simulink model "wzorzec_nasze"  (R2021b)
settings: Solver=ode5  StartTime=0.0  StopTime=20  FixedStep=0.01  RelTol=1e-3
settings Model: SimulationMode=external  ExtModeTrigDuration=100000  Creator=STUDENT  LastModifiedBy=STUDENT
settings SolverCC: AlgebraicLoopSolver=TrustRegion  DecoupledContinuousIntegration=on  MinimalZcImpactIntegration=on
settings DataIOCC: ReturnWorkspaceOutputs=off
settings DebuggingCC: PregeneratedLibrarySubsystemCodeDiagnostic=none  SFMachineParentedDataDiag=warning  ArithmeticOperatorsInVariantConditions=warning
settings SFSimCC: SimUseLocalCustomCode=off  CustomCodeUndefinedFunction=UseInterfaceOnly
settings RTWCC: Description=Simulink Desktop Real-Time  SystemTargetFile=sldrt.tlc  TemplateMakefile=sldrt.tmf  RTWUseLocalCustomCode=off  RTWCompilerOptimization=on
settings CodeAppCC: MaxIdLength=95
settings SimulinkDesktopRealTimeCC: TargetPreCompLibLocation=C:\apps\MATLAB\R2021b\toolbox\sldrt\lib\win64

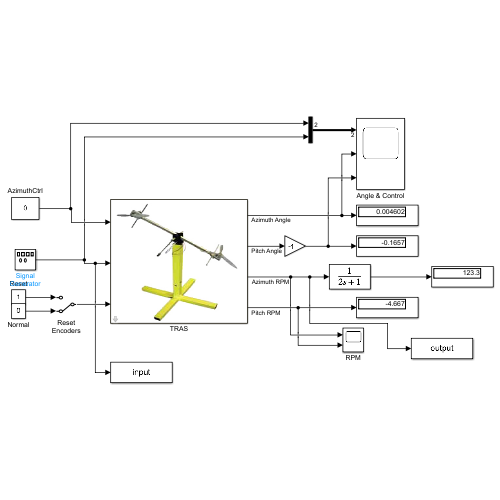
[thumbnail: Simulink's stored preview of the top-level diagram]
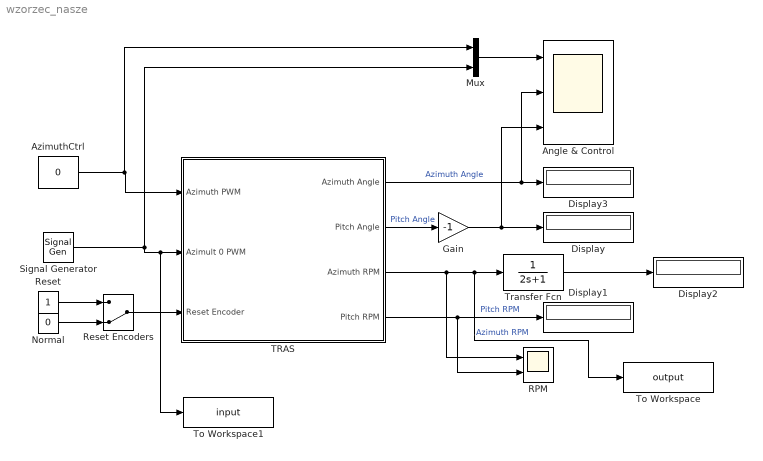
== system wzorzec_nasze ==
  Angle & Control : Scope  NumInputPorts=3
  AzimuthCtrl : Constant  Value=0
  Display{,1..3} (4 alike) : Display
  Gain : Gain  Gain=-1
  Mux : Mux  Inputs=2
  Normal : Constant  Value=0
  RPM : Scope  NumInputPorts=2
  Reset : Constant
  Reset Encoders : ManualSwitch  CurrentSetting=0
  Signal Generator : SignalGenerator  WaveForm=square  Amplitude=0.6  Frequency=0.5
  TRAS : Subsystem  mask{BaseAddress=57088, T0=0.01}
      mask prompts: BaseAddress "Base Address:"; T0 "Sampling Period:"
      mask Display: image('TRAS.JPG')
  To Workspace : ToWorkspace  VariableName=output  SaveFormat=Structure With Time  SampleTime=0.01
  To Workspace1 : ToWorkspace  VariableName=input  SaveFormat=Structure With Time  SampleTime=0.01
  Transfer Fcn : TransferFcn  Denominator=[2 1]
  wires:
  Reset/1 -> Reset Encoders/1
  TRAS/3(Azimuth RPM) -> To Workspace/1, Transfer Fcn/1, RPM/1  "Azimuth RPM"
  TRAS/1(Azimuth Angle) -> Angle & Control/2, Display3/1  "Azimuth Angle"
  TRAS/4(Pitch RPM) -> RPM/2, Display1/1  "Pitch RPM"
  Normal/1 -> Reset Encoders/2
  Reset Encoders/1 -> TRAS/3(Reset Encoder)
  TRAS/2(Pitch Angle) -> Gain/1  "Pitch Angle"
  Gain/1 -> Angle & Control/3, Display/1
  Mux/1 -> Angle & Control/1
  AzimuthCtrl/1 -> Mux/1, TRAS/1(Azimuth PWM)
  Transfer Fcn/1 -> Display2/1
  Signal Generator/1 -> To Workspace1/1, TRAS/2(Azimult 0 PWM), Mux/2

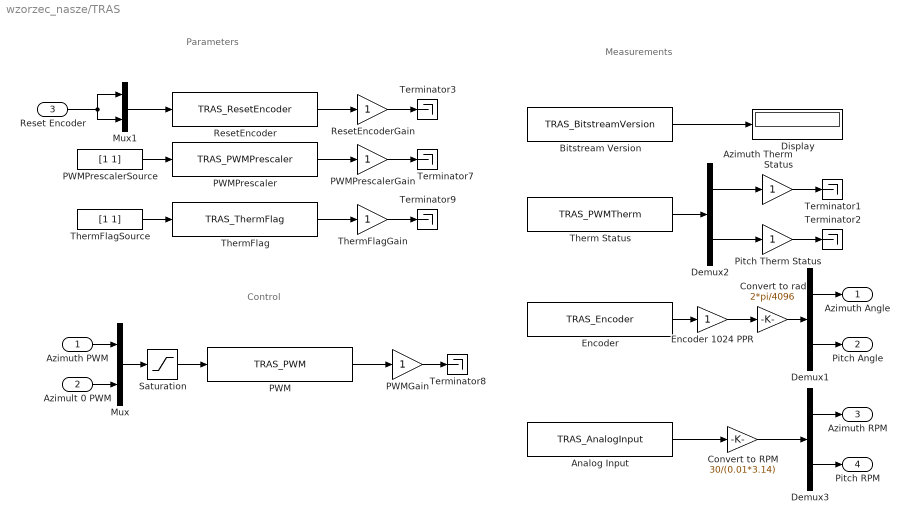
== system wzorzec_nasze/TRAS ==
  note: Parameters
  note: Control
  note: Measurements
  Azimuth PWM : Inport
  Azimult 0 PWM : Inport  Port=2
  Reset Encoder : Inport  Port=3
  Analog Input : S-Function  FunctionName=TRAS_AnalogInput  Parameters=BaseAddress, [1 0], [1 1], T0  SFunctionDeploymentMode=off  EnableBusSupport=off
  Azimuth Therm Status : Gain  SaturateOnIntegerOverflow=on  OutDataTypeStr=Inherit: Same as input  ParamDataTypeStr=Inherit: Same as input
  Bitstream Version : S-Function  FunctionName=TRAS_BitstreamVersion  Parameters=BaseAddress, T0  SFunctionDeploymentMode=off  EnableBusSupport=off
  Convert to RPM : Gain  Gain=30/(0.01*3.14)  SaturateOnIntegerOverflow=on  OutDataTypeStr=Inherit: Same as input  ParamDataTypeStr=Inherit: Same as input
  Convert to rad : Gain  Gain=2*pi/4096  SaturateOnIntegerOverflow=on  OutDataTypeStr=Inherit: Same as input  ParamDataTypeStr=Inherit: Same as input
  Demux1 : Demux  Outputs=2
      settings: DisplayOption=none
  Demux2 : Demux  Outputs=2
      settings: DisplayOption=none
  Demux3 : Demux  Outputs=2
      settings: DisplayOption=none
  Display : Display
  Encoder : S-Function  FunctionName=TRAS_Encoder  Parameters=BaseAddress, T0  SFunctionDeploymentMode=off  EnableBusSupport=off
  Encoder 1024 PPR : Gain  SaturateOnIntegerOverflow=on  OutDataTypeStr=Inherit: Same as input  ParamDataTypeStr=Inherit: Same as input
  Mux : Mux  Inputs=2
  Mux1 : Mux  Inputs=2
  PWM : S-Function  FunctionName=TRAS_PWM  Parameters=BaseAddress, T0  SFunctionDeploymentMode=off  EnableBusSupport=off
  PWMGain : Gain  SaturateOnIntegerOverflow=on  OutDataTypeStr=Inherit: Same as input  ParamDataTypeStr=Inherit: Same as input
  PWMPrescaler : S-Function  FunctionName=TRAS_PWMPrescaler  Parameters=BaseAddress, T0  SFunctionDeploymentMode=off  EnableBusSupport=off
  PWMPrescalerGain : Gain  SaturateOnIntegerOverflow=on  OutDataTypeStr=Inherit: Same as input  ParamDataTypeStr=Inherit: Same as input
  PWMPrescalerSource : Constant  Value=[1 1]
  Pitch Therm Status : Gain  SaturateOnIntegerOverflow=on  OutDataTypeStr=Inherit: Same as input  ParamDataTypeStr=Inherit: Same as input
  ResetEncoder : S-Function  FunctionName=TRAS_ResetEncoder  Parameters=BaseAddress, T0  SFunctionDeploymentMode=off  EnableBusSupport=off
  ResetEncoderGain : Gain  SaturateOnIntegerOverflow=on  OutDataTypeStr=Inherit: Same as input  ParamDataTypeStr=Inherit: Same as input
  Saturation : Saturate  UpperLimit=1  LowerLimit=-1
  Terminator{1..3,7..9} (6 alike) : Terminator
  Therm Status : S-Function  FunctionName=TRAS_PWMTherm  Parameters=BaseAddress, T0  SFunctionDeploymentMode=off  EnableBusSupport=off
  "ThermFlag " : S-Function  FunctionName=TRAS_ThermFlag  Parameters=BaseAddress, T0  SFunctionDeploymentMode=off  EnableBusSupport=off
  ThermFlagGain : Gain  SaturateOnIntegerOverflow=on  OutDataTypeStr=Inherit: Same as input  ParamDataTypeStr=Inherit: Same as input
  ThermFlagSource : Constant  Value=[1 1]
  Azimuth Angle : Outport  VectorParamsAs1DForOutWhenUnconnected=off
  Pitch Angle : Outport  Port=2  VectorParamsAs1DForOutWhenUnconnected=off
  Azimuth RPM : Outport  Port=3  VectorParamsAs1DForOutWhenUnconnected=off
  Pitch RPM : Outport  Port=4  VectorParamsAs1DForOutWhenUnconnected=off
  wires:
  Encoder 1024 PPR/1 -> Convert to rad/1
  Encoder/1 -> Encoder 1024 PPR/1
  Saturation/1 -> PWM/1
  Mux/1 -> Saturation/1
  PWM/1 -> PWMGain/1
  PWMGain/1 -> Terminator8/1
  ResetEncoder/1 -> ResetEncoderGain/1
  PWMPrescaler/1 -> PWMPrescalerGain/1
  Mux1/1 -> ResetEncoder/1
  PWMPrescalerSource/1 -> PWMPrescaler/1
  ResetEncoderGain/1 -> Terminator3/1
  PWMPrescalerGain/1 -> Terminator7/1
  Azimult 0 PWM/1 -> Mux/2
  Azimuth PWM/1 -> Mux/1
  Demux1/2 -> Pitch Angle/1
  Convert to rad/1 -> Demux1/1
  Demux1/1 -> Azimuth Angle/1
  Therm Status/1 -> Demux2/1
  Demux2/2 -> Pitch Therm Status/1
  Demux2/1 -> Azimuth Therm Status/1
  Azimuth Therm Status/1 -> Terminator1/1
  Pitch Therm Status/1 -> Terminator2/1
  Bitstream Version/1 -> Display/1
  Analog Input/1 -> Convert to RPM/1
  Demux3/2 -> Pitch RPM/1
  Demux3/1 -> Azimuth RPM/1
  Reset Encoder/1 -> Mux1/1, Mux1/2
  Convert to RPM/1 -> Demux3/1
  "ThermFlag "/1 -> ThermFlagGain/1
  ThermFlagSource/1 -> "ThermFlag "/1
  ThermFlagGain/1 -> Terminator9/1
